simulink model "Model_3_Hieu_1_12"  (R2021a)
settings: Solver=VariableStepAuto  StartTime=0.0  StopTime=10  RelTol=1e-3
InitFcn:
  | ml=0.2;
  | mc=0.5;
  | mt=0.5;
  | g=9.81;
  | l_ref=0.5;
  | l_ini=0.5;
  | l=l_ini;
  | n1=5;n2=1;
  | x_ref=10;
  | 
  | %ADRC' s parameter caculation
  | %b0 = (ml+mc)/(mc*ml +mc*mt+ml*mt); %Hieu
  | b0=(ml+mc)/(mt*mc+2*ml*mc+mt*ml+ml^2+mc^2); %Enhanced-coupling
  | k_ESO = 50;
  | T_set  = 6;
  | 
  | s_cl = -5.85/T_set;
  | Kp   = s_cl^2;
  | Kd   = -2*s_cl;
  | 
  | s_ESO = k_ESO*s_cl;
  | l1        = -3*s_ESO;
  | l2        = 3*( s_ESO)^2;
  | l3        = -(s_ESO)^3;
  | 
  | %Observer
  | A = [-l1, 1, 0;
  |         -l2, 0, 1;
  |         -l3, 0, 0];
  | B = [0;
  |         b0;
  |         0];
  | L = [l1;
  |        l2;
  |        l3];
  | 
  | %b1 = (mt+mc)/(mc*ml +mc*mt+ml*mt);
  | b1=1/(ml+mc);
  | k_ESO1 =100;
  | T_set1  = 3;
  | s_cl1 = -5.85/T_set1;
  | Kp1   = s_cl1^2;
  | Kd1   = -2*s_cl1;
  | 
  | s_ESO1 = k_ESO1*s_cl1;
  | l11        = -3*s_ESO1;
  | l21        = 3*( s_ESO1)^2;
  | l31        = -(s_ESO1)^3;
  | 
  | %Observer
  | A1 = [-l11, 1, 0;
  |         -l21, 0, 1;
  |         -l31, 0, 0];
  | B1 = [0;
  |         b1;
  |         0];
  | L1 = [l11;
  |        l21;
  |        l31];
  | 
  | ... (+35 lines)
values from neighbouring files (symbols this model uses):
  particle = repmat(empty_particle, nPop, 1)    [PSO16_12.m]    (also in PSO_ZVD.m)
undefined symbols (not defined in the file or in its folder): i
libraries: neural x35, simulink_extras x11, simulink x5
(part 11 of 15)

== matlab function Model_3_Hieu_1_12/Heiu/Model_Baocao/Crane ==
  data: d1x input; l input; d1l input; the input; dx1 output; d1the input; Fx input; Fl input; dx2 output; dx3 output; dx4 output; dx5 output; dx6 output; bc input; mp input
function [dx1,dx2,dx3,dx4,dx5,dx6] = fcn(d1x,l,d1l,the,d1the,Fx,Fl,bc,mp)
 mt =5; mh =2; bt =20; br =50;  g =9.81;

dx1 = d1x;
dx2 = (Fx*l*mh + Fx*l*mp - Fl*l*mp*sin(the) + bc*d1the*mh*cos(the) + bc*d1the*mp*cos(the) - d1the^2*l^2*mp^2*sin(the) + d1x^2*l^2*mp^2*sin(the) - bt*d1x*l*mh - bt*d1x*l*mp + d1x^2*l^2*mh*mp*sin(the) + br*d1l*l*mp*sin(the) + g*l*mh*mp*cos(the)*sin(the))/(l*(mh*mp + mh*mt + mp*mt - mp^2*cos(the)^2 - mp^2*sin(the)^2 + mp^2 - mh*mp*cos(the)^2));
%dx2= -(bt*x2*mc - ml*ut - mc*ul*sin(x5) - mc*ut + bt*x2*ml - x6^2*x3*mc^2*sin(x5) + br*x4*mc*sin(x5) + Dt*x6*mc^2*cos(x5) + x6^2*x3*mc*ml*sin(x5) + g*mc*ml*cos(x5)*sin(x5) + Dt*x6*mc*ml*cos(x5))/(mc*ml + mc*mt + ml*mt - mc^2*cos(x5)^2 - mc^2*sin(x5)^2 + mc^2 - mc*ml*cos(x5)^2);
 
dx3 = d1l;
dx4 = -(d1x^2*l^2*mp^2*sin(the)^2 - Fl*l*mt - d1the^2*l^2*mp^2 - Fl*l*mp + g*l*mp^2*cos(the)^3 + Fx*l*mp*sin(the) + Fl*l*mp*cos(the)^2 - d1the^2*l^2*mp*mt - g*l*mp^2*cos(the) + d1the^2*l^2*mp^2*cos(the)^2 + br*d1l*l*mp + br*d1l*l*mt + g*l*mp^2*cos(the)*sin(the)^2 - br*d1l*l*mp*cos(the)^2 + bc*d1the*mp*cos(the)*sin(the) - g*l*mp*mt*cos(the) - bt*d1x*l*mp*sin(the))/(l*(mh*mp + mh*mt + mp*mt - mp^2*cos(the)^2 - mp^2*sin(the)^2 + mp^2 - mh*mp*cos(the)^2));
%dx4 = -(mc*ul*cos(x5)^2 - mt*ul - mc*ut*sin(x5) - 2*x6^2*x3*mc^2 - g*mc^2*cos(x5) - mc*ul + br*x4*mc + br*x4*mt + g*mc^2*cos(x5)^3 - 2*x6^2*x3*mc*mt - g*mc*mt*cos(x5) + bt*x2*mc*sin(x5) + 2*x6^2*x3*mc^2*cos(x5)^2 + x6^2*x3*mc^2*sin(x5)^2 + g*mc^2*cos(x5)*sin(x5)^2 - br*x4*mc*cos(x5)^2 + Dt*x6*mc^2*cos(x5)*sin(x5))/(mc*ml + mc*mt + ml*mt - mc^2*cos(x5)^2 - mc^2*sin(x5)^2 + mc^2 - mc*ml*cos(x5)^2);
dx5 = d1the;
dx6 = -(bc*d1the*mp^2 + bc*d1the*mh*mp + bc*d1the*mh*mt + bc*d1the*mp*mt - bc*d1the*mp^2*sin(the)^2 - g*l*mp^3*sin(the)^3 + 2*d1l*d1the*l*mp^3 + Fx*l*mp^2*cos(the) + g*l*mp^3*sin(the) - g*l*mp^3*cos(the)^2*sin(the) - bt*d1x*l*mp^2*cos(the) + g*l*mh*mp^2*sin(the) + g*l*mp^2*mt*sin(the) - d1the^2*l^2*mp^3*cos(the)*sin(the) + d1x^2*l^2*mp^3*cos(the)*sin(the) - 2*d1l*d1the*l*mp^3*cos(the)^2 - Fl*l*mp^2*cos(the)*sin(the) - 2*d1l*d1the*l*mp^3*sin(the)^2 + Fx*l*mh*mp*cos(the) + 2*d1l*d1the*l*mh*mp^2 + 2*d1l*d1the*l*mp^2*mt - 2*d1l*d1the*l*mh*mp^2*cos(the)^2 + br*d1l*l*mp^2*cos(the)*sin(the) - bt*d1x*l*mh*mp*cos(the) + g*l*mh*mp*mt*sin(the) + 2*d1l*d1the*l*mh*mp*mt + d1x^2*l^2*mh*mp^2*cos(the)*sin(the))/(l^2*mp*(mh*mp + mh*mt + mp*mt - mp^2*cos(the)^2 - mp^2*sin(the)^2 + mp^2 - mh*mp*cos(the)^2));
%dx6 = -(g*mc^2*sin(x5) - ml*ut*cos(x5) - mc*ut*cos(x5) + Dt*x6*mc^2 - g*mc^2*sin(x5)^3 + 2*x4*x6*mc^2 - mc*ul*cos(x5)*sin(x5) + 2*x4*x6*mc*ml + 2*x4*x6*mc*mt + 2*x4*x6*ml*mt - Dt*x6*mc^2*sin(x5)^2 - 2*x4*x6*mc^2*cos(x5)^2 - 2*x4*x6*mc^2*sin(x5)^2 + bt*x2*mc*cos(x5) + bt*x2*ml*cos(x5) + g*mc*ml*sin(x5) + g*mc*mt*sin(x5) + g*ml*mt*sin(x5) - g*mc^2*cos(x5)^2*sin(x5) + Dt*x6*mc*ml + Dt*x6*mc*mt + Dt*x6*ml*mt - x6^2*x3*mc^2*cos(x5)*sin(x5) - 2*x4*x6*mc*ml*cos(x5)^2 + br*x4*mc*cos(x5)*sin(x5) + x6^2*x3*mc*ml*cos(x5)*sin(x5))/(x3*(mc*ml + mc*mt + ml*mt - mc^2*cos(x5)^2 - mc^2*sin(x5)^2 + mc^2 - mc*ml*cos(x5)^2));
